simulink model "lab2_MC_integration"  (Simulink 8.9)
settings: Solver=ode3  StartTime=0.0  StopTime=5000.0  FixedStep=1  RelTol=1e-3  EnableMultiTasking=on
undefined symbols (not defined in the file): DiscIntNeverNeededParam
settings Model: Creator=IEUser  LastModifiedBy=igorkislyuk
settings OptimizationCC: BooleanDataType=off  ExpressionDepthLimit=2147483647
settings DebuggingCC: SolverPrmCheckMsg=warning
settings GRTTargetCC: GeneratePreprocessorConditionals=Use local settings

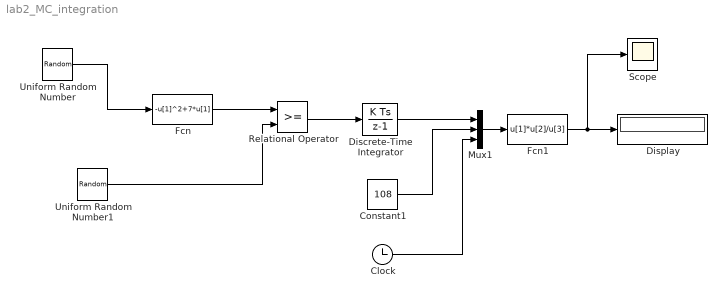
== system lab2_MC_integration ==
  Clock : Clock
  Constant1 : Constant  Value=108
  Discrete-Time Integrator : DiscreteIntegrator  OutDataTypeStr=double  ICPrevOutput=DiscIntNeverNeededParam  ICPrevScaledInput=DiscIntNeverNeededParam
  Display : Display
  Fcn : Fcn  Expr=-u[1]^2+7*u[1]
  Fcn1 : Fcn  Expr=u[1]*u[2]/u[3]
  Mux1 : Mux  Inputs=3
  Relational Operator : RelationalOperator  OutDataTypeStr=boolean  RndMeth=Nearest
  Scope : Scope
  Uniform Random Number : UniformRandomNumber  Minimum=-6  Maximum=10  Seed=5  SampleTime=0
  Uniform Random Number1 : UniformRandomNumber  Minimum=0  Maximum=8  SampleTime=0
  wires:
  Fcn/1 -> Relational Operator/1
  Relational Operator/1 -> Discrete-Time Integrator/1
  Discrete-Time Integrator/1 -> Mux1/1
  Constant1/1 -> Mux1/2
  Clock/1 -> Mux1/3
  Mux1/1 -> Fcn1/1
  Fcn1/1 -> Display/1, Scope/1
  Uniform Random Number/1 -> Fcn/1
  Uniform Random Number1/1 -> Relational Operator/2
